simulink model "sdd_model"  (R2020b)
settings: Solver=ode4  StartTime=0.0  StopTime=10  FixedStep=modelStep  MaxStep=1e-5  RelTol=1e-3
values from neighbouring files (symbols this model uses):
  Bh = [Bx_h1, By_h1, Bz_h1] + [Bx_h2, By_h2, Bz_h2]    [config.m]
  degX0 = 0    [config.m]
  degZ0 = 0    [config.m]
  frictionCoef = 0.00001    (= 1e-05)    [config.m]
  frictionLinearCoef = 1    [config.m]
  frictionQuadraticCoef = 0.001    [config.m]
  StructModelConst = 15378.18722131129492333262    (= 15378.1872213)    [config.m]
  VZ0 = 0    [config.m]
undefined symbols (not defined in the file or in its folder): custom_pwm, pwm, sigbuilder_block
libraries: fl_lib x10, nesl_utility x6, simulink x2, pid_lib x1
settings Model: TunableVars=Disbalance,StructModelConst,VX0,VZ0,degX0,degZ0,frictionCoef,frictionLinearCoef,frictionQuadraticCoef  TunableVarsStorageClass=Auto,Auto,Auto,Auto,Auto,Auto,Auto,Auto,Auto  TunableVarsTypeQualifier=,,,,,,,,  OrderedModelArguments=off  Creator=nrx  LastModifiedBy=nrx
settings SolverCC: ZeroCrossControl=DisableAll  ZeroCrossAlgorithm=Adaptive
settings DataIOCC: SaveState=on  InspectSignalLogs=on
settings OptimizationCC: UseDivisionForNetSlopeComputation=on  GainParamInheritBuiltInType=on  UseFloatMulNetSlope=on  StrengthReduction=on  PassReuseOutputArgsThreshold=0  ZeroExternalMemoryAtStartup=off  ZeroInternalMemoryAtStartup=off  EfficientFloat2IntCast=on  OptimizeBlockOrder=speed  OptimizationPriority=Speed  OptimizationCustomize=off  MultiThreadedLoops=on
settings DebuggingCC: ParameterTunabilityLossMsg=error
settings HardwareCC: ProdBitPerLong=64  ProdHWDeviceType=Intel->x86-64 (Linux 64)
settings SFSimCC: MATLABDynamicMemAlloc=off  SimTargetLang=C++
settings RTWCC: GenCodeOnly=on  PackageGeneratedCodeAndArtifacts=on  PackageName=sdd  GenerateReport=on  BuildConfiguration=Faster Runs  LaunchReport=on  TargetLang=C++
settings CodeAppCC: ForceParamTrailComments=on  OperatorAnnotations=on
settings GRTTargetCC: TargetLangStandard=C++03 (ISO)  CodeInterfacePackaging=C++ class  MultiInstanceErrorCode=Warning

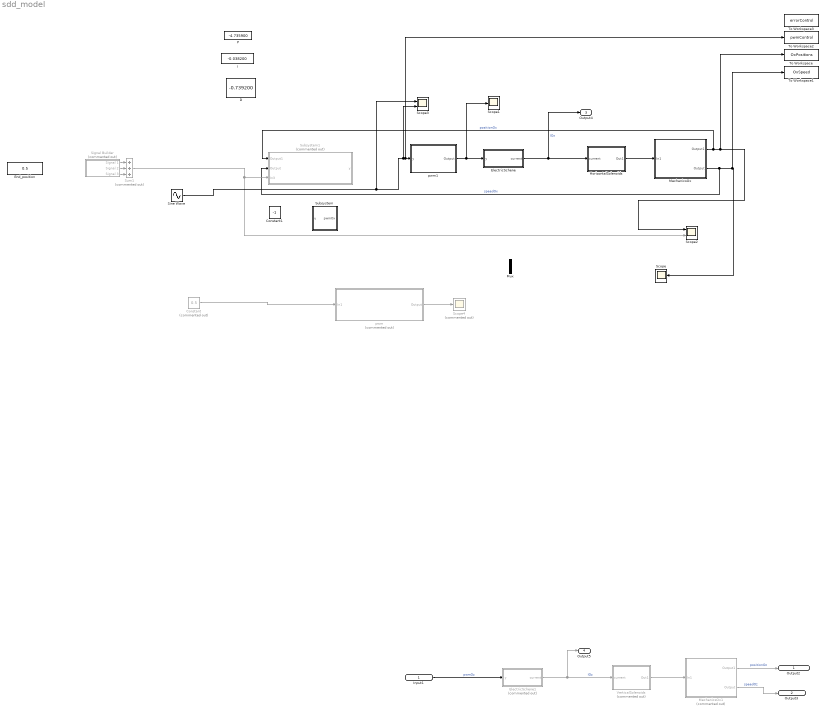
== system sdd_model ==
  Input1 : Inport
  Constant : Constant  Commented=on  Value=0.5
  Constant1 : Constant  Value=-1
  D : Constant  Value=-0.739200
  ElectricSchene : Subsystem
  ElectricSchene1 : Subsystem  Commented=on
  End_position : Constant  Value=0.5
  HorizontalSolenoids : Subsystem
  I : Constant  Value=-0.038200
  MechanicsOx : Subsystem
  MechanicsOx1 : Subsystem  Commented=on
  Mux : Mux  Inputs=2
  P : Constant  Value=-4.735900
  Scope : Scope
  Scope1 : Scope
  Scope2 : Scope  NumInputPorts=2
  Scope3 : Scope  NumInputPorts=2
  Scope4 : Scope  Commented=on
  Signal Builder : Subsystem  Tag=STV Subsys  Commented=on  LoadFcn=sigbuilder_block('load');  StartFcn=sigbuilder_block('start');  StopFcn=sigbuilder_block('stop');  ClipboardFcn=sigbuilder_block('clipboard');  mask(Sigbuilder block){tuvar=[0:10]}
      mask help: Simulink:masks:SigbuilderBlock_MD
      mask init:
      | if ~strcmp(get_param(bdroot(gcbh),'SimulationStatus'),'stopped') tuvar = sigbuilder_block('maskInit'); end
      settings: CopyFcn=sigbuilder_block('copy');  DeleteFcn=sigbuilder_block('delete');  ModelCloseFcn=sigbuilder_block('modelClose');  PreSaveFcn=sigbuilder_block('preSave');  PauseFcn=sigbuilder_block('pause');  ContinueFcn=sigbuilder_block('continue');  NameChangeFcn=sigbuilder_block('namechange');  OpenFcn=sigbuilder_block('open',[429.75 192 565.5 399.75 ]);  CloseFcn=sigbuilder_block('close');
      mask Display: plot(0, 0, 100, 100,[2, 2, 32, 32, 2], [68, 8, 8, 68, 68],[32, 2], [38, 38], [32, 19, 2],[53, 60, 44], [32, 17, 17, 2],[16, 16, 31, 31]);txt = getActiveGroup(gcbh);text(2, 100, txt,'verticalAlignment', 'top');
  Sine Wave : Sin  Frequency=10  Phase=pi/2  SampleTime=0
  Subsystem : Subsystem
  Subsystem1 : Subsystem  Commented=on
  Sum1 : Sum  Commented=on  Inputs=+++
  To Workspace : ToWorkspace  VariableName=OxPositions  SampleTime=1/100
      settings: Save2DSignal=2-D array (concatenate along first dimension)
  To Workspace1 : ToWorkspace  VariableName=OxSpeed  SampleTime=1/100
  To Workspace2 : ToWorkspace  VariableName=pwmControl  SampleTime=1/100
      settings: Save2DSignal=2-D array (concatenate along first dimension)
  To Workspace3 : ToWorkspace  VariableName=errorControl  SampleTime=1/100
      settings: Save2DSignal=2-D array (concatenate along first dimension)
  VerticalSolenoids : Subsystem  Commented=on
  pwm : Subsystem  Commented=on  AncestorBlock=custom_pwm/pwm
  pwm1 : Subsystem  AncestorBlock=custom_pwm/pwm
  Output2 : Outport  SignalName=positionOz
  Output3 : Outport  Port=2  SignalName=speedOz
  Output4 : Outport  Port=3  SignalName=IOx
  Output5 : Outport  Port=4  SignalName=IOz
  wires:
  ElectricSchene/1(current) -> Output4/1, HorizontalSolenoids/1(current)  "IOx"
  ElectricSchene1/1(current) -> Output5/1, VerticalSolenoids/1(current)  "IOz"
  MechanicsOx/1(Output1) -> Subsystem1/1(Output1), To Workspace/1, Scope2/1  "positionOx"
  MechanicsOx/2(Output) -> Subsystem1/2(Output), To Workspace1/1, Scope/1  "speedOx"
  Input1/1 -> ElectricSchene1/1(y)  "pwmOz"
  MechanicsOx1/1(Output1) -> Output2/1  "positionOz"
  MechanicsOx1/2(Output) -> Output3/1  "speedOz"
  HorizontalSolenoids/1(Out1) -> MechanicsOx/1(In1)
  VerticalSolenoids/1(Out1) -> MechanicsOx1/1(In1)
  Constant/1 -> pwm/1(In1)
  pwm/1(Output) -> Scope4/1
  pwm1/1(Output) -> Scope1/1, ElectricSchene/1(y)
  Signal Builder/1(Signal 1) -> Sum1/1
  Signal Builder/2(Signal 2) -> Sum1/2
  Signal Builder/3(Signal 3) -> Sum1/3
  Sum1/1 -> Scope2/2, Subsystem1/3(In3)
  Sine Wave/1 -> Scope3/1, Scope3/2, To Workspace2/1, pwm1/1(y)

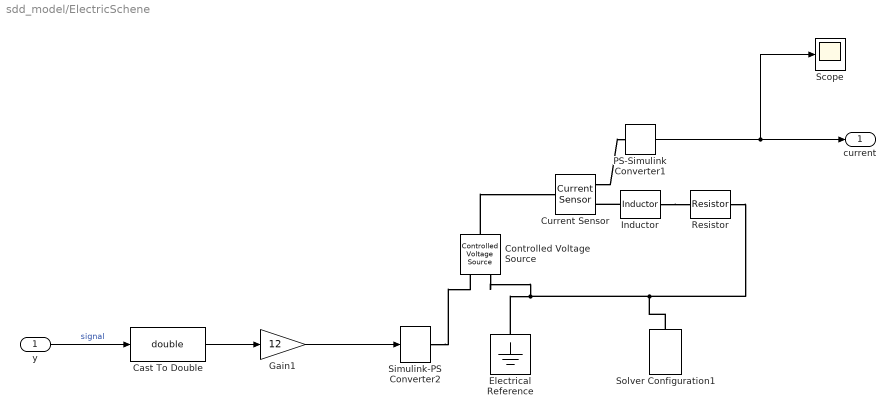
== system sdd_model/ElectricSchene ==
  y : Inport
  Cast To Double : DataTypeConversion  OutDataTypeStr=double
  Controlled Voltage Source : fl_lib/Electrical/Electrical Sources/Controlled Voltage Source
  Current Sensor : fl_lib/Electrical/Electrical Sensors/Current Sensor
  Electrical Reference : fl_lib/Electrical/Electrical Elements/Electrical Reference
  Gain1 : Gain  Gain=12
  Inductor : fl_lib/Electrical/Electrical Elements/Inductor  l=909.038 uH  r=0 Ohm  g=1e-9 1/Ohm  i_specify=off  i_priority=High  i=0 A  i_nominal_specify=off  i_nominal_unit=A  i_nominal_value=1  v_specify=off  v_priority=High  v=0 V  v_nominal_specify=off  v_nominal_unit=V  v_nominal_value=1  i_L_specify=off  i_L_priority=High  i_L=0 A  i_L_nominal_specify=off  i_L_nominal_unit=A  i_L_nominal_value=1
  PS-Simulink Converter1 : nesl_utility/PS-Simulink Converter  PhysicalDomain=network_engine_domain  SubClassName=ps_output  LeftPortType=input  RightPortType=output  PseudoPeriodic=off  Frequencies=[]  Unit=A  AffineConversion=off
  Resistor : fl_lib/Electrical/Electrical Elements/Resistor  R=4 Ohm  i_specify=off  i_priority=High  i=0 A  i_nominal_specify=off  i_nominal_unit=A  i_nominal_value=1  v_specify=off  v_priority=High  v=0 V  v_nominal_specify=off  v_nominal_unit=V  v_nominal_value=1
  Scope : Scope
  Simulink-PS Converter2 : nesl_utility/Simulink-PS Converter  PhysicalDomain=network_engine_domain  SubClassName=ps_input  LeftPortType=input  RightPortType=output  PseudoPeriodic=off  Frequencies=[]  NoiseDistribution=none  NoiseParameters=[]  Unit=1  AffineConversion=off  FilteringAndDerivatives=zero  SimscapeFilterOrder=1  InputFilterTimeConstant=0.001  UdotUserProvided=1
  Solver Configuration1 : nesl_utility/Solver Configuration  PhysicalDomain=network_engine_domain  SubClassName=solver  LeftPortType=input  RightPortType=generic  Tones=[]  Harmonics=[]  SimulateNoise=off  Profile=off  UseLocalSampling=off  EnableSwitchedLinearOptims=on  FrequencyDomain=off  UseCCode=off  RelTol=0.001  AbsTol=1e-06  MinStep=1e-09  ToWorkspace=off  RevertToSquareIcSolve=off  NumHomotopyIterations=100  PhasorMode=off  PhasorModeNumHarmonics=1  DoDC=off  ResidualTolerance=1e-03  UseLocalSolver=off  LocalSolverChoice=NE_BACKWARD_EULER_ADVANCER  LocalSolverSampleTime=0.001  DoFixedCost=off  MaxNonlinIter=3  MaxModeIter=2  ComputeImpulses=off  ImpulseIterations=2  LinearAlgebra=Sparse  EquationFormulation=NE_TIME_EF  DelaysMemoryBudget=1024  AutomaticFiltering=on  FilteringTimeConstant=0.001  PartitionStorageMethod=AS_NEEDED  PartitionMemoryBudget=1024  PartitionMethod=FAST
  current : Outport  VectorParamsAs1DForOutWhenUnconnected=off
  wires:
  PS-Simulink Converter1/1 -> Scope/1, current/1
  Gain1/1 -> Simulink-PS Converter2/1
  Cast To Double/1 -> Gain1/1
  y/1 -> Cast To Double/1  "signal"
  connections:
  Solver Configuration1/RConn1 -- Resistor/RConn1 -- Electrical Reference/LConn1 -- Controlled Voltage Source/RConn2
  Controlled Voltage Source/LConn1 -- Current Sensor/LConn1
  Inductor/LConn1 -- Current Sensor/RConn2
  Inductor/RConn1 -- Resistor/LConn1
  Current Sensor/RConn1 -- PS-Simulink Converter1/LConn1
  Simulink-PS Converter2/RConn1 -- Controlled Voltage Source/RConn1

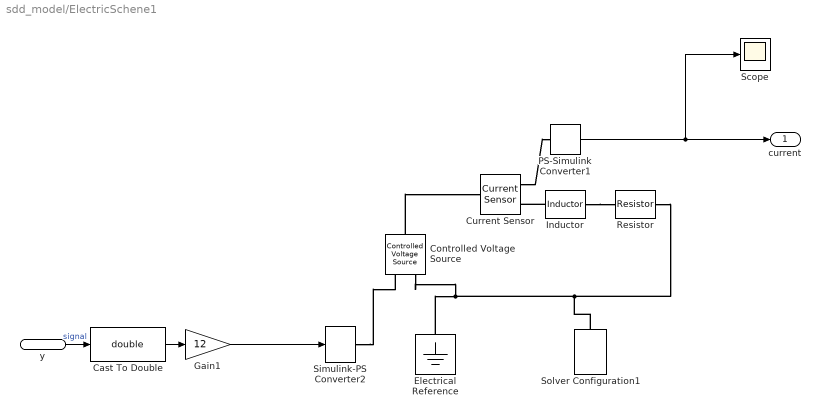
== system sdd_model/ElectricSchene1 ==
  y : Inport
  Cast To Double : DataTypeConversion  OutDataTypeStr=double
  Controlled Voltage Source : fl_lib/Electrical/Electrical Sources/Controlled Voltage Source
  Current Sensor : fl_lib/Electrical/Electrical Sensors/Current Sensor
  Electrical Reference : fl_lib/Electrical/Electrical Elements/Electrical Reference
  Gain1 : Gain  Gain=12
  Inductor : fl_lib/Electrical/Electrical Elements/Inductor  l=909.038 uH  r=0 Ohm  g=1e-9 1/Ohm  i_specify=off  i_priority=High  i=0 A  i_nominal_specify=off  i_nominal_unit=A  i_nominal_value=1  v_specify=off  v_priority=High  v=0 V  v_nominal_specify=off  v_nominal_unit=V  v_nominal_value=1  i_L_specify=off  i_L_priority=High  i_L=0 A  i_L_nominal_specify=off  i_L_nominal_unit=A  i_L_nominal_value=1
  PS-Simulink Converter1 : nesl_utility/PS-Simulink Converter  PhysicalDomain=network_engine_domain  SubClassName=ps_output  LeftPortType=input  RightPortType=output  PseudoPeriodic=off  Frequencies=[]  Unit=A  AffineConversion=off
  Resistor : fl_lib/Electrical/Electrical Elements/Resistor  R=4 Ohm  i_specify=off  i_priority=High  i=0 A  i_nominal_specify=off  i_nominal_unit=A  i_nominal_value=1  v_specify=off  v_priority=High  v=0 V  v_nominal_specify=off  v_nominal_unit=V  v_nominal_value=1
  Scope : Scope
  Simulink-PS Converter2 : nesl_utility/Simulink-PS Converter  PhysicalDomain=network_engine_domain  SubClassName=ps_input  LeftPortType=input  RightPortType=output  PseudoPeriodic=off  Frequencies=[]  NoiseDistribution=none  NoiseParameters=[]  Unit=1  AffineConversion=off  FilteringAndDerivatives=zero  SimscapeFilterOrder=1  InputFilterTimeConstant=0.001  UdotUserProvided=1
  Solver Configuration1 : nesl_utility/Solver Configuration  PhysicalDomain=network_engine_domain  SubClassName=solver  LeftPortType=input  RightPortType=generic  Tones=[]  Harmonics=[]  SimulateNoise=off  Profile=off  UseLocalSampling=off  EnableSwitchedLinearOptims=on  FrequencyDomain=off  UseCCode=off  RelTol=0.001  AbsTol=1e-06  MinStep=1e-09  ToWorkspace=off  RevertToSquareIcSolve=off  NumHomotopyIterations=100  PhasorMode=off  PhasorModeNumHarmonics=1  DoDC=off  ResidualTolerance=1e-03  UseLocalSolver=off  LocalSolverChoice=NE_BACKWARD_EULER_ADVANCER  LocalSolverSampleTime=0.001  DoFixedCost=off  MaxNonlinIter=3  MaxModeIter=2  LinearAlgebra=Sparse  EquationFormulation=NE_TIME_EF  DelaysMemoryBudget=1024  AutomaticFiltering=on  FilteringTimeConstant=0.001  PartitionStorageMethod=AS_NEEDED  PartitionMemoryBudget=1024  PartitionMethod=FAST
  current : Outport  VectorParamsAs1DForOutWhenUnconnected=off
  wires:
  PS-Simulink Converter1/1 -> Scope/1, current/1
  Gain1/1 -> Simulink-PS Converter2/1
  y/1 -> Cast To Double/1  "signal"
  Cast To Double/1 -> Gain1/1
  connections:
  Solver Configuration1/RConn1 -- Resistor/RConn1 -- Electrical Reference/LConn1 -- Controlled Voltage Source/RConn2
  Controlled Voltage Source/LConn1 -- Current Sensor/LConn1
  Inductor/LConn1 -- Current Sensor/RConn2
  Inductor/RConn1 -- Resistor/LConn1
  Current Sensor/RConn1 -- PS-Simulink Converter1/LConn1
  Simulink-PS Converter2/RConn1 -- Controlled Voltage Source/RConn1

== system sdd_model/HorizontalSolenoids ==
  current : Inport
  BHorizontal : Constant  Value=Bh
  Product : Product
  Out1 : Outport
  wires:
  BHorizontal/1 -> Product/1
  current/1 -> Product/2  "I"
  Product/1 -> Out1/1

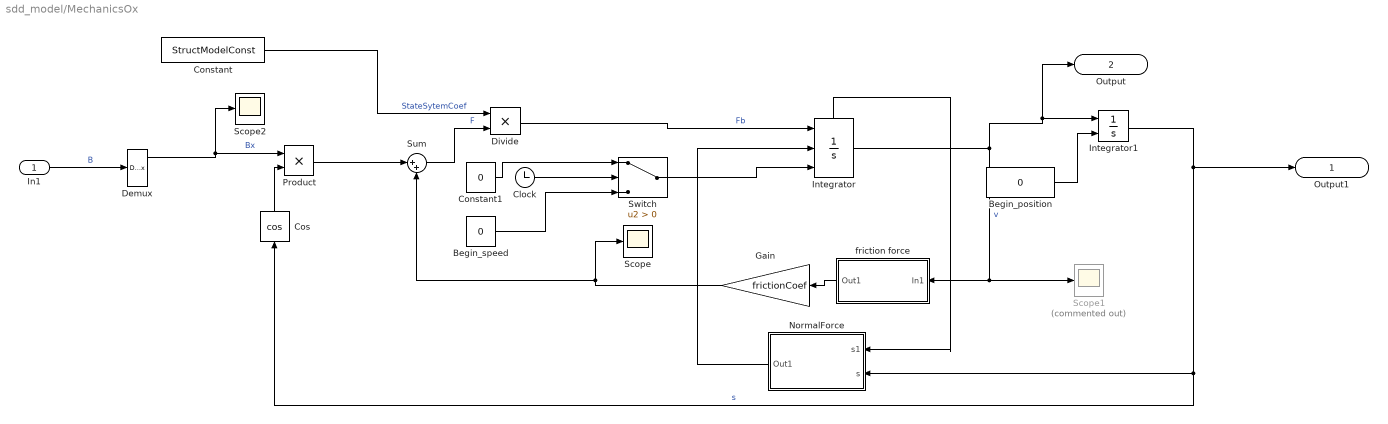
== system sdd_model/MechanicsOx ==
  In1 : Inport
  Begin_position : Constant  Value=0
  Begin_speed : Constant  Value=0
  Clock : Clock
  Constant : Constant  Value=StructModelConst
  Constant1 : Constant  Value=0
  Cos : Trigonometry  Operator=cos
  Demux : Demux  Outputs=3
  Divide : Product  Inputs=**
  Gain : Gain  Gain=frictionCoef
  Integrator : Integrator  ExternalReset=level  InitialConditionSource=external  ShowStatePort=on
  Integrator1 : Integrator  InitialConditionSource=external  InitialCondition=degX0
  NormalForce : Subsystem
  Product : Product
  Scope : Scope
  Scope1 : Scope  Commented=on
  Scope2 : Scope
  Sum : Sum  Inputs=|++
  Switch : Switch  Criteria=u2 > Threshold
  friction force : Subsystem
  Output1 : Outport
  Output : Outport  Port=2
  wires:
  Product/1 -> Sum/1
  Demux/1 -> Product/1, Scope2/1  "Bx"
  Integrator/1 -> Output/1, Integrator1/1, friction force/1(In1), Scope1/1  "v"
  In1/1 -> Demux/1  "B"
  Cos/1 -> Product/2
  Gain/1 -> Scope/1, Sum/2
  NormalForce/1(Out1) -> Integrator/2
  friction force/1(Out1) -> Gain/1
  Integrator1/1 -> Output1/1, NormalForce/2(s), Cos/1  "s"
  Sum/1 -> Divide/2  "F"
  Integrator/State -> NormalForce/1(s1)
  Divide/1 -> Integrator/1  "Fb"
  Constant/1 -> Divide/1  "StateSytemCoef"
  Clock/1 -> Switch/2
  Constant1/1 -> Switch/1
  Begin_speed/1 -> Switch/3
  Switch/1 -> Integrator/3
  Begin_position/1 -> Integrator1/2

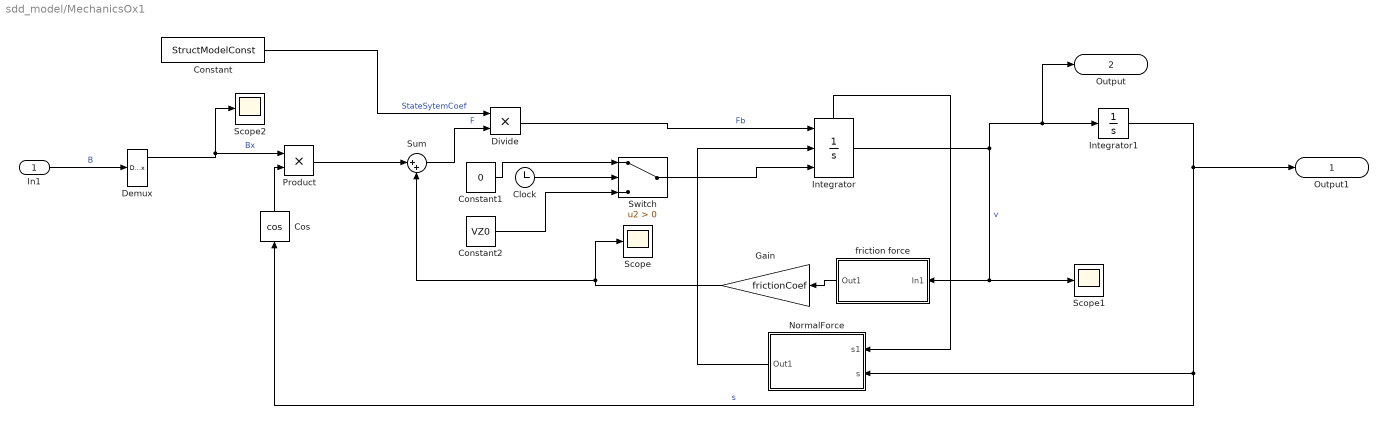
== system sdd_model/MechanicsOx1 ==
  In1 : Inport
  Clock : Clock
  Constant : Constant  Value=StructModelConst
  Constant1 : Constant  Value=0
  Constant2 : Constant  Value=VZ0
  Cos : Trigonometry  Operator=cos
  Demux : Demux  Outputs=3
  Divide : Product  Inputs=**
  Gain : Gain  Gain=frictionCoef
  Integrator : Integrator  ExternalReset=level  InitialConditionSource=external  ShowStatePort=on
  Integrator1 : Integrator  InitialCondition=degZ0
  NormalForce : Subsystem
  Product : Product
  Scope : Scope
  Scope1 : Scope
  Scope2 : Scope
  Sum : Sum  Inputs=|++
  Switch : Switch  Criteria=u2 > Threshold
  friction force : Subsystem
  Output1 : Outport
  Output : Outport  Port=2
  wires:
  Product/1 -> Sum/1
  Demux/1 -> Product/1, Scope2/1  "Bx"
  Integrator/1 -> Output/1, Integrator1/1, friction force/1(In1), Scope1/1  "v"
  In1/1 -> Demux/1  "B"
  Cos/1 -> Product/2
  Gain/1 -> Scope/1, Sum/2
  NormalForce/1(Out1) -> Integrator/2
  friction force/1(Out1) -> Gain/1
  Integrator1/1 -> Output1/1, NormalForce/2(s), Cos/1  "s"
  Sum/1 -> Divide/2  "F"
  Integrator/State -> NormalForce/1(s1)
  Divide/1 -> Integrator/1  "Fb"
  Constant/1 -> Divide/1  "StateSytemCoef"
  Clock/1 -> Switch/2
  Constant1/1 -> Switch/1
  Constant2/1 -> Switch/3
  Switch/1 -> Integrator/3

== system sdd_model/Signal Builder ==
  Demux : Demux  Tag=STV Demux  Outputs=3
      settings: DisplayOption=none
  FromWs : FromWorkspace  Tag=STV FromWs  VariableName=tuvar
      SigBuilderData=|
      | common.afterFinalStr = 'Extrapolate'
      | common.sampleTime = 0
      | dataSet.timeRange = [0 10]
      | dataSet.name = 'Group 1'
      | sbobj.Groups.Name = 'Group 1'
      | sbobj.Groups.Signals(1).Name = 'Signal 1'
      | sbobj.Groups.Signals(1).XData = [0 0.08 0.08 1 1 10]
      | sbobj.Groups.Signals(1).YData = [0 0 0.5 0.5 0 0]
      | sbobj.Groups.Signals(2).Name = 'Signal 2'
      | sbobj.Groups.Signals(2).XData = [0 1.9 1.9 2.58 2.58 10]
      | sbobj.Groups.Signals(2).YData = [0 0 -0.5 -0.5 0 0]
      | sbobj.Groups.Signals(3).Name = 'Signal 3'
      | sbobj.Groups.Signals(3).XData = [0 2.64 2.64 3.18 3.18 10]
      | sbobj.Groups.Signals(3).YData = [0 0 0.5 0.5 0 0]
  Signal 1 : Outport  Tag=STV Outport
  Signal 2 : Outport  Tag=STV Outport  Port=2
  Signal 3 : Outport  Tag=STV Outport  Port=3
  wires:
  Demux/1 -> Signal 1/1
  FromWs/1 -> Demux/1
  Demux/2 -> Signal 2/1
  Demux/3 -> Signal 3/1

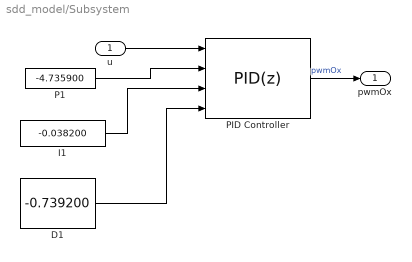
== system sdd_model/Subsystem ==
  u : Inport
  D1 : Constant  Value=-0.739200
  I1 : Constant  Value=-0.038200
  P1 : Constant  Value=-4.735900
  PID Controller : pid_lib/PID Controller  Controller=PID  Form=Parallel  TimeDomain=Discrete-time  UseExternalTs=off  SampleTime=1/100  IntegratorMethod=Forward Euler  FilterMethod=Forward Euler  ControllerParametersSource=external  P=-1.2  I=-1.85  D=-0.3  UseFilter=off  N=100  TunerSelectOption=Transfer Function Based (PID Tuner App)  InitialConditionSource=internal  InitialConditionForIntegrator=0  InitialConditionForFilter=0  DifferentiatorICPrevScaledInput=0  ExternalReset=none  TrackingMode=off  Kt=1  LimitOutput=on  SatLimitsSource=internal  UpperSaturationLimit=1  LowerSaturationLimit=-1  LinearizeAsGain=on  AntiWindupMode=none  Kb=1  POutMin=[]  POutMax=[]  IOutMin=[]  IOutMax=[]  DOutMin=[]  DOutMax=[]  NOutMin=[]  NOutMax=[]  SumOutMin=[]  SumOutMax=[]  SaturationOutMin=[]  SaturationOutMax=[]  PParamMin=[]  PParamMax=[]  IParamMin=[]  IParamMax=[]  DParamMin=[]  DParamMax=[]  NParamMin=[]  NParamMax=[]  KbParamMin=[]  KbParamMax=[]  KtParamMin=[]  KtParamMax=[]  KbOutMin=[]  KbOutMax=[]  KtOutMin=[]  KtOutMax=[]  IntegratorOutMin=[]  IntegratorOutMax=[]  FilterOutMin=[]  FilterOutMax=[]  SumI1OutMin=[]  SumI1OutMax=[]  SumI2OutMin=[]  SumI2OutMax=[]  SumI3OutMin=[]  SumI3OutMax=[]  SumI4OutMin=[]  SumI4OutMax=[]  SumDOutMin=[]  SumDOutMax=[]  DifferentiatorOutMin=[]  DifferentiatorOutMax=[]  FilterDiffOutCoefMin=[]  FilterDiffOutCoefMax=[]  ReciprocalOutMin=[]  ReciprocalOutMax=[]  SumDenOutMin=[]  SumDenOutMax=[]  SumNumOutMin=[]  SumNumOutMax=[]  DivideOutMin=[]  DivideOutMax=[]  UdiffTsProdOutMin=[]  UdiffTsProdOutMax=[]  NTsProdOutMin=[]  NTsProdOutMax=[]  UintegralTsProdOutMin=[]  UintegralTsProdOutMax=[]  UngainTsProdOutMin=[]  UngainTsProdOutMax=[]  IntegratorContinuousStateAttributes=''  IntegratorStateMustResolveToSignalObject=off  IntegratorRTWStateStorageClass=Auto  FilterContinuousStateAttributes=''  FilterStateMustResolveToSignalObject=off  FilterRTWStateStorageClass=Auto  ParallelPVariant=ExternalParameters  IdealPVariant=Disabled  IVariant=ExternalParameters  DVariant=ExternalParameters  IntegratorVariant=Discrete  SatVariant=Enabled  AWVariant=Passthrough  PCopyVariant=Disabled  TRVariant=Disabled  FdbkBlocksVariant=Forward  IdealPFdbkVariant=Disabled  SatFdbkVariant=Disabled  DerivativeFilterVariant=Differentiator  NVariant=Passthrough  NCopyVariant=Disabled_SignalSpec  FilterICVariant=InternalICsDifferentiator  IntegratorICVariant=InternalICs  ExternalResetVariant=Disabled  TRSumVariant=Passthrough  SumFdbkVariant=Disabled  SumVariant=Sum_PID  TsampFilterVariant=InternalTs  TsampNgainVariant=Passthrough  TsampIntegralVariant=Passthrough  ExternalSaturationOutDataTypeStr=Inherit: Same as second input
  pwmOx : Outport
  wires:
  P1/1 -> PID Controller/2
  I1/1 -> PID Controller/3
  D1/1 -> PID Controller/4
  u/1 -> PID Controller/1
  PID Controller/1 -> pwmOx/1  "pwmOx"

== system sdd_model/Subsystem1 ==
  Output1 : Inport
  Output : Inport  Port=2
  In3 : Inport  Port=3
  S-Function : S-Function  FunctionName=neurla_http_client_sfunc  Parameters=3  SFunctionDeploymentMode=off  EnableBusSupport=off
  y : Outport
  wires:
  S-Function/1 -> y/1  "duty_cycle"
  In3/1 -> S-Function/3  "end_pos"
  Output/1 -> S-Function/2  "ox_speed"
  Output1/1 -> S-Function/1  "ox_pos"

== system sdd_model/VerticalSolenoids ==
  current : Inport
  BHorizontal : Constant  Value=Bh
  Product : Product
  Out1 : Outport
  wires:
  BHorizontal/1 -> Product/1
  current/1 -> Product/2  "I"
  Product/1 -> Out1/1

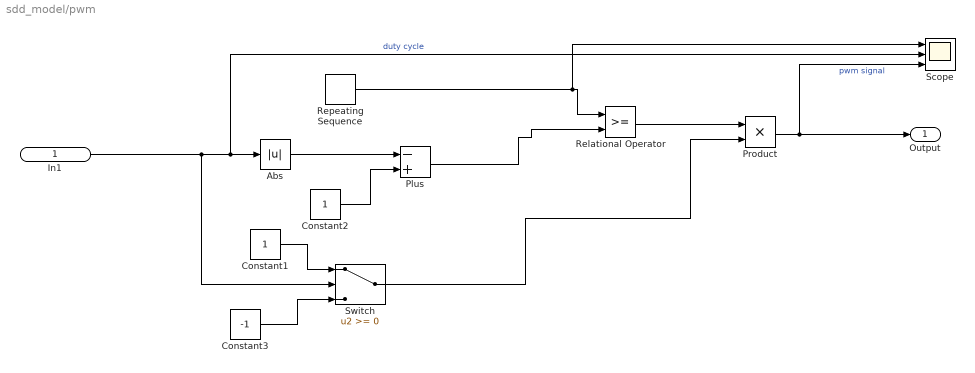
== system sdd_model/pwm ==
  In1 : Inport
  Abs : Abs
  Constant1 : Constant
  Constant2 : Constant
  Constant3 : Constant  Value=-1
  Plus : Sum  Inputs=-+
  Product : Product
  Relational Operator : RelationalOperator  OutDataTypeStr=boolean  RndMeth=Simplest
  Repeating Sequence : simulink/Sources/Repeating Sequence  rep_seq_t=[0 1]*1/100  rep_seq_y=[1 0]
  Scope : Scope  NumInputPorts=3
  Switch : Switch
  Output : Outport
  wires:
  Constant3/1 -> Switch/3
  Constant1/1 -> Switch/1
  Switch/1 -> Product/2
  Abs/1 -> Plus/1
  Product/1 -> Scope/3, Output/1  "pwm signal"
  Plus/1 -> Relational Operator/2
  Constant2/1 -> Plus/2
  In1/1 -> Abs/1, Scope/2, Switch/2  "duty cycle"
  Relational Operator/1 -> Product/1
  Repeating Sequence/1 -> Relational Operator/1, Scope/1

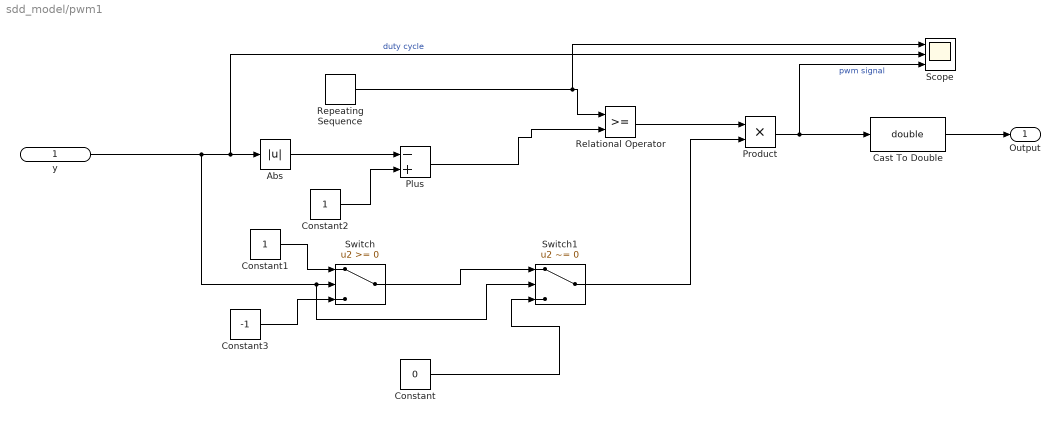
== system sdd_model/pwm1 ==
  y : Inport
  Abs : Abs
  Cast To Double : DataTypeConversion  OutDataTypeStr=double
  Constant : Constant  Value=0
  Constant1 : Constant
  Constant2 : Constant
  Constant3 : Constant  Value=-1
  Plus : Sum  Inputs=-+
  Product : Product
  Relational Operator : RelationalOperator  OutDataTypeStr=boolean  RndMeth=Simplest
  Repeating Sequence : simulink/Sources/Repeating Sequence  rep_seq_t=[0 1]*1/100  rep_seq_y=[1 0]
  Scope : Scope  NumInputPorts=3
  Switch : Switch
  Switch1 : Switch  Criteria=u2 ~= 0
  Output : Outport
  wires:
  Constant3/1 -> Switch/3
  Constant1/1 -> Switch/1
  Switch/1 -> Switch1/1
  Abs/1 -> Plus/1
  Product/1 -> Cast To Double/1, Scope/3  "pwm signal"
  Plus/1 -> Relational Operator/2
  Constant2/1 -> Plus/2
  y/1 -> Abs/1, Scope/2, Switch1/2, Switch/2  "duty cycle"
  Relational Operator/1 -> Product/1
  Repeating Sequence/1 -> Relational Operator/1, Scope/1
  Cast To Double/1 -> Output/1
  Constant/1 -> Switch1/3
  Switch1/1 -> Product/2

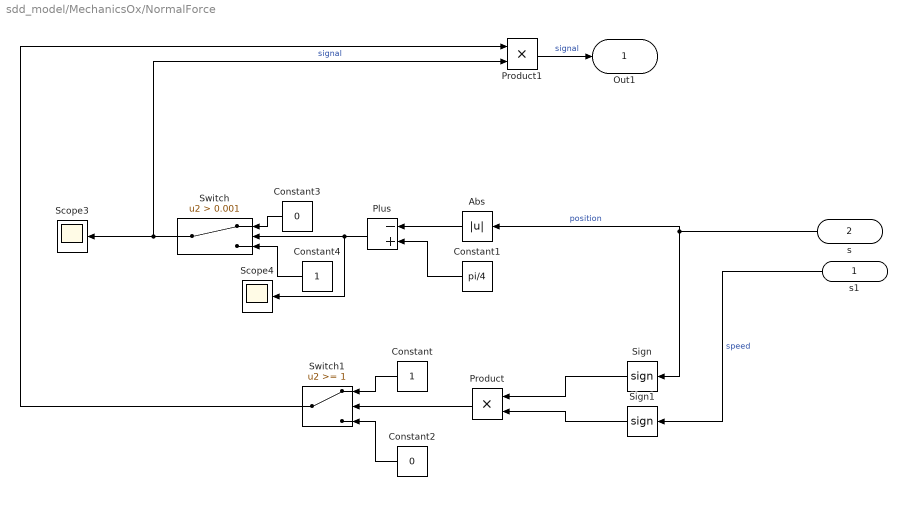
== system sdd_model/MechanicsOx/NormalForce ==
  s1 : Inport
  s : Inport  Port=2
  Abs : Abs
  Constant : Constant
  Constant1 : Constant  Value=pi/4
  Constant2 : Constant  Value=0
  Constant3 : Constant  Value=0
  Constant4 : Constant
  Plus : Sum  Inputs=-+
  Product : Product
  Product1 : Product
  Scope3 : Scope
  Scope4 : Scope
  Sign : Signum
  Sign1 : Signum
  Switch : Switch  Criteria=u2 > Threshold  Threshold=0.001
  Switch1 : Switch  Threshold=1
  Out1 : Outport
  wires:
  Constant1/1 -> Plus/2
  s/1 -> Abs/1, Sign/1  "position"
  Abs/1 -> Plus/1
  Constant4/1 -> Switch/3
  Plus/1 -> Scope4/1, Switch/2
  Switch/1 -> Product1/2, Scope3/1  "signal"
  Constant3/1 -> Switch/1
  s1/1 -> Sign1/1  "speed"
  Sign/1 -> Product/1
  Sign1/1 -> Product/2
  Product/1 -> Switch1/2
  Constant/1 -> Switch1/1
  Constant2/1 -> Switch1/3
  Product1/1 -> Out1/1  "signal"
  Switch1/1 -> Product1/1

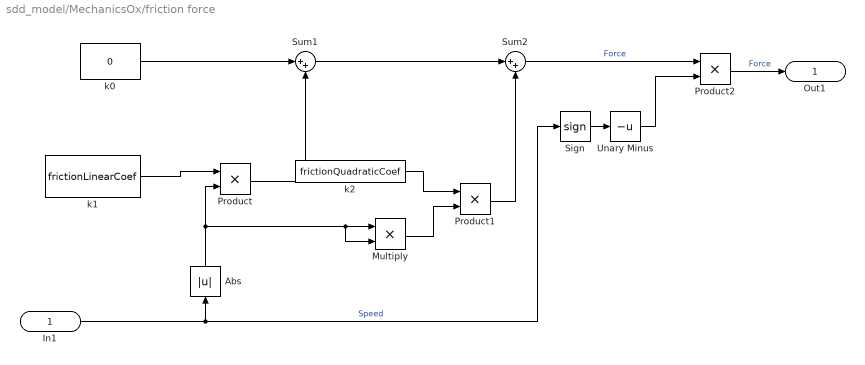
== system sdd_model/MechanicsOx/friction force ==
  In1 : Inport
  Abs : Abs
  Multiply : Product
  Product : Product
  Product1 : Product
  Product2 : Product
  Sign : Signum
  Sum1 : Sum  Inputs=|++
  Sum2 : Sum  Inputs=|++
  Unary Minus : UnaryMinus
  k0 : Constant  Value=0
  k1 : Constant  Value=frictionLinearCoef
  k2 : Constant  Value=frictionQuadraticCoef
  Out1 : Outport
  wires:
  Sum2/1 -> Product2/1  "Force"
  k1/1 -> Product/1
  Multiply/1 -> Product1/2
  k0/1 -> Sum1/1
  k2/1 -> Product1/1
  In1/1 -> Sign/1, Abs/1  "Speed"
  Product/1 -> Sum1/2
  Sum1/1 -> Sum2/1
  Product1/1 -> Sum2/2
  Abs/1 -> Multiply/2, Multiply/1, Product/2
  Sign/1 -> Unary Minus/1
  Product2/1 -> Out1/1  "Force"
  Unary Minus/1 -> Product2/2

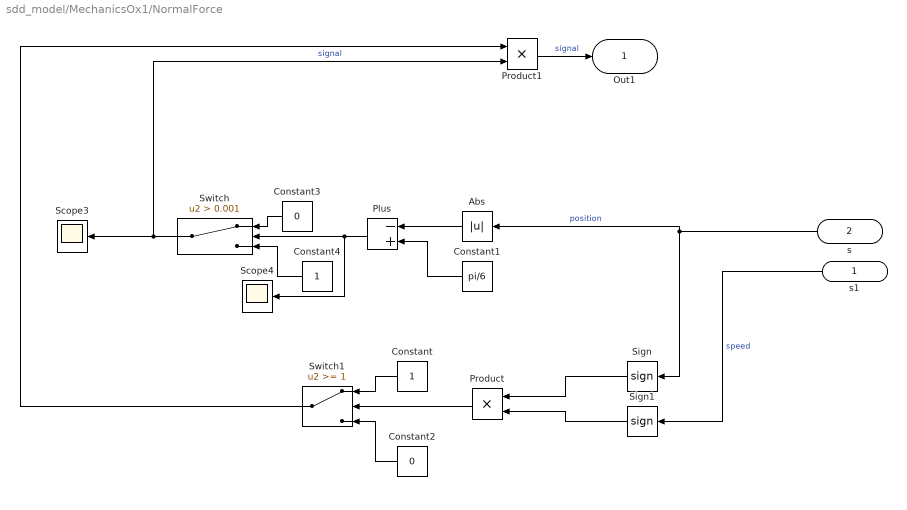
== system sdd_model/MechanicsOx1/NormalForce ==
  s1 : Inport
  s : Inport  Port=2
  Abs : Abs
  Constant : Constant
  Constant1 : Constant  Value=pi/6
  Constant2 : Constant  Value=0
  Constant3 : Constant  Value=0
  Constant4 : Constant
  Plus : Sum  Inputs=-+
  Product : Product
  Product1 : Product
  Scope3 : Scope
  Scope4 : Scope
  Sign : Signum
  Sign1 : Signum
  Switch : Switch  Criteria=u2 > Threshold  Threshold=0.001
  Switch1 : Switch  Threshold=1
  Out1 : Outport
  wires:
  Constant1/1 -> Plus/2
  s/1 -> Abs/1, Sign/1  "position"
  Abs/1 -> Plus/1
  Constant4/1 -> Switch/3
  Plus/1 -> Scope4/1, Switch/2
  Switch/1 -> Product1/2, Scope3/1  "signal"
  Constant3/1 -> Switch/1
  s1/1 -> Sign1/1  "speed"
  Sign/1 -> Product/1
  Sign1/1 -> Product/2
  Product/1 -> Switch1/2
  Constant/1 -> Switch1/1
  Constant2/1 -> Switch1/3
  Product1/1 -> Out1/1  "signal"
  Switch1/1 -> Product1/1

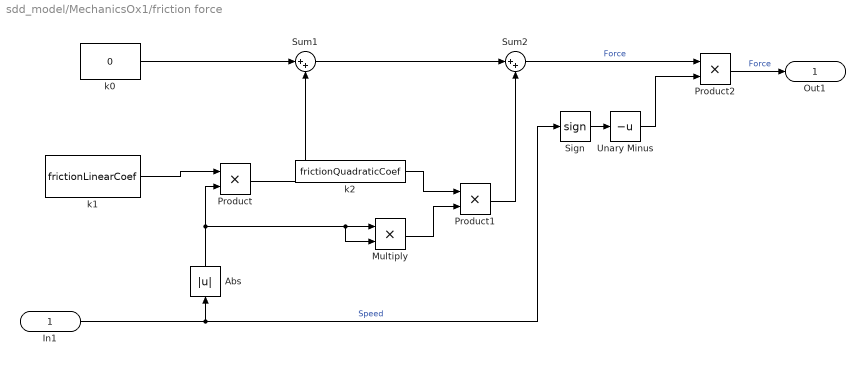
== system sdd_model/MechanicsOx1/friction force ==
  In1 : Inport
  Abs : Abs
  Multiply : Product
  Product : Product
  Product1 : Product
  Product2 : Product
  Sign : Signum
  Sum1 : Sum  Inputs=|++
  Sum2 : Sum  Inputs=|++
  Unary Minus : UnaryMinus
  k0 : Constant  Value=0
  k1 : Constant  Value=frictionLinearCoef
  k2 : Constant  Value=frictionQuadraticCoef
  Out1 : Outport
  wires:
  Sum2/1 -> Product2/1  "Force"
  k1/1 -> Product/1
  Multiply/1 -> Product1/2
  k0/1 -> Sum1/1
  k2/1 -> Product1/1
  In1/1 -> Sign/1, Abs/1  "Speed"
  Product/1 -> Sum1/2
  Sum1/1 -> Sum2/1
  Product1/1 -> Sum2/2
  Abs/1 -> Multiply/2, Multiply/1, Product/2
  Sign/1 -> Unary Minus/1
  Product2/1 -> Out1/1  "Force"
  Unary Minus/1 -> Product2/2
